simulink model "VINS"  (R2018a)
settings: Solver=FixedStepDiscrete  StartTime=0.0  StopTime=inf  FixedStep=1/Fs  RelTol=1e-3  EnableMultiTasking=on
PreLoadFcn:
  | modelDef = getModelDef(calibrateSFMA);
  | 
  | %imuPar = getImuPar('lmvpUncalibrated');
  | 
  | timeMatchThreshold = 1000;
undefined symbols (not defined in the file or in its folder): beep, dejitter_on, Fs, homogeneous3x4Transform_k_kmin1, imuLocationMm, imuPar, numStates, simData, tstamp_k_us, tstamp_kmin1_us
libraries: simulink x69, dspmtrx3 x35, dspindex x9, vrlib x7, dspstat3 x7, dspinverses x6, dspsigops x5, dspmathops x2, rtwdemowidgets x1, dspfactors x1, simulink_extras x1
(part 2 of 6)

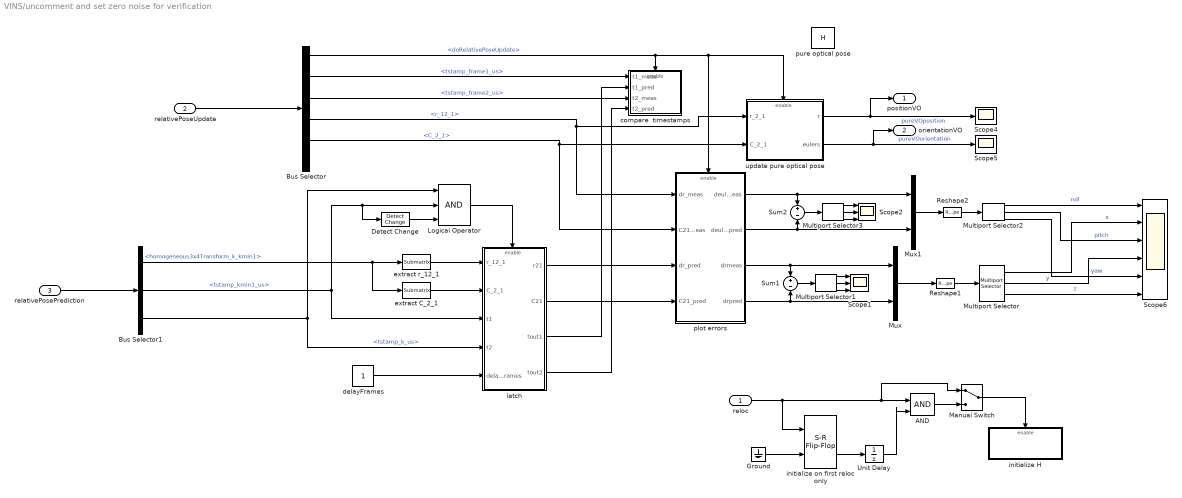
== system VINS/uncomment and set zero noise for verification ==
  reloc : Inport
  relativePoseUpdate : Inport  Port=2
  relativePosePrediction : Inport  Port=3
  AND : Logic  IconShape=distinctive  AllPortsSameDT=off  OutDataTypeStr=boolean
  Bus Selector : BusSelector  OutputSignals=doRelativePoseUpdate,tstamp_frame1_us,tstamp_frame2_us,r_12_1,C_2_1,poseErrorCovariance
  Bus Selector1 : BusSelector  OutputSignals=homogeneous3x4Transform_k_kmin1,tstamp_kmin1_us,tstamp_k_us
  Detect Change : simulink/Logic and Bit Operations/Detect Change  vinit=0  OutDataTypeStr=boolean
  Ground : Ground
  Logical Operator : Logic  Inputs=3  AllPortsSameDT=off  OutDataTypeStr=boolean
  Manual Switch : ManualSwitch
  Multiport Selector{,1..3} (4 alike) : dspindex/Multiport Selector  rowsOrCols=Rows  idxCellArray={1,2,3 }  idxErrMode=Clip Index
  Mux : Mux  Inputs=2
  Mux1 : Mux  Inputs=2
  Reshape1 : Reshape  OutputDimensionality=Customize  OutputDimensions=[3,2]
  Reshape2 : Reshape  OutputDimensionality=Customize  OutputDimensions=[3,2]
  Scope1 : Scope  NumInputPorts=3
  Scope2 : Scope  NumInputPorts=3
  Scope4 : Scope
  Scope5 : Scope
  Scope6 : Scope  NumInputPorts=6
  Sum1 : Sum  Inputs=+-
  Sum2 : Sum  Inputs=+-
  Unit Delay : UnitDelay  SampleTime=-1
  compare  timestamps : Subsystem  TreatAsAtomicUnit=on
  delayFrames : Constant
  extract C_2_1 : dspmtrx3/Submatrix  RowSpan=Range of rows  RowStartMode=First  RowStartIndex=1  RowEndMode=Index  RowEndIndex=3  ColSpan=Range of columns  ColStartMode=First  ColStartIndex=1  ColEndMode=Index  ColEndIndex=3
  extract r_12_1 : dspmtrx3/Submatrix  RowSpan=Range of rows  RowStartMode=First  RowStartIndex=1  RowEndMode=Index  RowEndIndex=3  ColSpan=One column  ColStartMode=Last  ColStartIndex=1  ColEndMode=Index  ColEndIndex=3
  initialize H : Subsystem  TreatAsAtomicUnit=on
  initialize on first reloc only : simulink_extras/Flip Flops/S-R Flip-Flop  initial_condition=0
  latch : Subsystem  TreatAsAtomicUnit=on
  plot errors : Subsystem  TreatAsAtomicUnit=on
  pure optical pose : DataStoreMemory  DataStoreName=H  ReadBeforeWriteMsg=warning  WriteAfterWriteMsg=warning  WriteAfterReadMsg=warning  InitialValue=eye(4)  ShowAdditionalParam=off
  update pure optical pose : Subsystem  TreatAsAtomicUnit=on
  positionVO : Outport
  orientationVO : Outport  Port=2
  wires:
  relativePoseUpdate/1 -> Bus Selector/1
  Bus Selector/1 -> plot errors/Enable, update pure optical pose/Enable, compare  timestamps/Enable  "<doRelativePoseUpdate>"
  Bus Selector/4 -> update pure optical pose/1(r_2_1), plot errors/1(dr_meas)  "<r_12_1>"
  Bus Selector/5 -> plot errors/2(C21_meas), update pure optical pose/2(C_2_1)  "<C_2_1>"
  relativePosePrediction/1 -> Bus Selector1/1
  Bus Selector1/1 -> extract C_2_1/1, extract r_12_1/1  "<homogeneous3x4Transform_k_kmin1>"
  Bus Selector/2 -> compare  timestamps/1(t1_meas)  "<tstamp_frame1_us>"
  Bus Selector/3 -> compare  timestamps/3(t2_meas)  "<tstamp_frame2_us>"
  extract r_12_1/1 -> latch/1(r_12_1)
  extract C_2_1/1 -> latch/2(C_2_1)
  Bus Selector1/3 -> latch/4(t2), Logical Operator/1  "<tstamp_k_us>"
  Bus Selector1/2 -> latch/3(t1), Detect Change/1, Logical Operator/2  "<tstamp_kmin1_us>"
  Logical Operator/1 -> latch/Enable
  latch/3(tout1) -> compare  timestamps/2(t1_pred)
  latch/4(tout2) -> compare  timestamps/4(t2_pred)
  latch/1(r21) -> plot errors/3(dr_pred)
  latch/2(C21) -> plot errors/4(C21_pred)
  plot errors/4(drpred) -> Mux/2, Sum1/2
  plot errors/3(drmeas) -> Mux/1, Sum1/1
  Sum1/1 -> Multiport Selector1/1
  delayFrames/1 -> latch/5(delayFrames)
  Detect Change/1 -> Logical Operator/3
  update pure optical pose/1(r) -> Scope4/1, positionVO/1  "pureVOposition"
  update pure optical pose/2(eulers) -> orientationVO/1, Scope5/1  "pureVOorientation"
  Mux/1 -> Reshape1/1
  Reshape1/1 -> Multiport Selector/1
  Multiport Selector1/3 -> Scope1/3
  Multiport Selector1/1 -> Scope1/1
  Multiport Selector1/2 -> Scope1/2
  Multiport Selector3/2 -> Scope2/2
  Multiport Selector3/1 -> Scope2/1
  Multiport Selector3/3 -> Scope2/3
  Reshape2/1 -> Multiport Selector2/1
  Mux1/1 -> Reshape2/1
  Sum2/1 -> Multiport Selector3/1
  plot errors/1(deul_meas) -> Sum2/1, Mux1/1
  plot errors/2(deul_pred) -> Sum2/2, Mux1/2
  Multiport Selector2/1 -> Scope6/1  "roll"
  Multiport Selector/1 -> Scope6/2  "x"
  Multiport Selector2/2 -> Scope6/3  "pitch"
  Multiport Selector/2 -> Scope6/4  "y"
  Multiport Selector2/3 -> Scope6/5  "yaw"
  Multiport Selector/3 -> Scope6/6  "z"
  reloc/1 -> initialize on first reloc only/1, Manual Switch/1, AND/1
  Manual Switch/1 -> initialize H/Enable
  initialize on first reloc only/2 -> Unit Delay/1
  Unit Delay/1 -> AND/2
  Ground/1 -> initialize on first reloc only/2
  AND/1 -> Manual Switch/2

== system VINS/INS/DT police ==
  In1 : Inport
  Data Store Read : DataStoreRead  DataStoreName=DataTypeRef
  Data Type Duplicate : DataTypeDuplicate
  wires:
  Data Store Read/1 -> Data Type Duplicate/1
  In1/1 -> Data Type Duplicate/2

== system VINS/augmentState/DT convert ==
  In1 : Inport
  Data Store Read : DataStoreRead  DataStoreName=DataTypeRef
  Data Type Conversion Inherited : simulink/Signal Attributes/Data Type Conversion Inherited  ConvertRealWorld=Real World Value  DoSatur=off
      settings: SourceProductName=Simulink  SourceProductBaseCode=SL
  Out1 : Outport
  wires:
  Data Type Conversion Inherited/1 -> Out1/1
  Data Store Read/1 -> Data Type Conversion Inherited/1
  In1/1 -> Data Type Conversion Inherited/2

== system VINS/augmentState/DT convert1 ==
  In1 : Inport
  Data Store Read : DataStoreRead  DataStoreName=DataTypeRef
  Data Type Conversion Inherited : simulink/Signal Attributes/Data Type Conversion Inherited  ConvertRealWorld=Real World Value  DoSatur=off
      settings: SourceProductName=Simulink  SourceProductBaseCode=SL
  Out1 : Outport
  wires:
  In1/1 -> Data Type Conversion Inherited/2
  Data Store Read/1 -> Data Type Conversion Inherited/1
  Data Type Conversion Inherited/1 -> Out1/1

== system VINS/augmentState/DT police1 ==
  In1 : Inport
  Data Store Read : DataStoreRead  DataStoreName=DataTypeRef
  Data Type Duplicate : DataTypeDuplicate
  wires:
  Data Store Read/1 -> Data Type Duplicate/1
  In1/1 -> Data Type Duplicate/2

== system VINS/augmentState/DT police2 ==
  In1 : Inport
  Data Store Read : DataStoreRead  DataStoreName=DataTypeRef
  Data Type Duplicate : DataTypeDuplicate
  wires:
  Data Store Read/1 -> Data Type Duplicate/1
  In1/1 -> Data Type Duplicate/2

== system VINS/augmentState/DT police3 ==
  In1 : Inport
  Data Store Read : DataStoreRead  DataStoreName=DataTypeRef
  Data Type Duplicate : DataTypeDuplicate
  wires:
  In1/1 -> Data Type Duplicate/2
  Data Store Read/1 -> Data Type Duplicate/1

== system VINS/augmentState/DT police4 ==
  In1 : Inport
  Data Store Read : DataStoreRead  DataStoreName=DataTypeRef
  Data Type Duplicate : DataTypeDuplicate
  wires:
  Data Store Read/1 -> Data Type Duplicate/1
  In1/1 -> Data Type Duplicate/2

== system VINS/augmentState/DT police5 ==
  In1 : Inport
  Data Store Read : DataStoreRead  DataStoreName=DataTypeRef
  Data Type Duplicate : DataTypeDuplicate
  wires:
  In1/1 -> Data Type Duplicate/2
  Data Store Read/1 -> Data Type Duplicate/1

== system VINS/augmentState/DT police6 ==
  In1 : Inport
  Data Store Read : DataStoreRead  DataStoreName=DataTypeRef
  Data Type Duplicate : DataTypeDuplicate
  wires:
  Data Store Read/1 -> Data Type Duplicate/1
  In1/1 -> Data Type Duplicate/2

== system VINS/augmentState/DT police7 ==
  In1 : Inport
  Data Store Read : DataStoreRead  DataStoreName=DataTypeRef
  Data Type Duplicate : DataTypeDuplicate
  wires:
  In1/1 -> Data Type Duplicate/2
  Data Store Read/1 -> Data Type Duplicate/1

== system VINS/augmentState/DT police8 ==
  In1 : Inport
  Data Store Read : DataStoreRead  DataStoreName=DataTypeRef
  Data Type Duplicate : DataTypeDuplicate
  wires:
  Data Store Read/1 -> Data Type Duplicate/1
  In1/1 -> Data Type Duplicate/2

== system VINS/augmentState/DT police9 ==
  In1 : Inport
  Data Store Read : DataStoreRead  DataStoreName=DataTypeRef
  Data Type Duplicate : DataTypeDuplicate
  wires:
  In1/1 -> Data Type Duplicate/2
  Data Store Read/1 -> Data Type Duplicate/1

== system VINS/augmentState/advancePoseIndex ==
  Bias : Bias  Bias=1
  Constant : Constant  Value=modelDef.maxNumDelayedPoses
  Data Store Read : DataStoreRead  DataStoreName=newestDelayedPoseIdx
  Data Store Write2 : DataStoreWrite  DataStoreName=newestDelayedPoseIdx
  Relational Operator : RelationalOperator  Operator=<=  OutDataTypeStr=boolean  RndMeth=Simplest
  Switch : Switch  Criteria=u2 > Threshold
  rollover back to one : Constant  Value=uint8(1)
  newIndex : Outport
  wires:
  Data Store Read/1 -> Bias/1
  Bias/1 -> Switch/1, Relational Operator/1
  Constant/1 -> Relational Operator/2
  Relational Operator/1 -> Switch/2
  Switch/1 -> newIndex/1, Data Store Write2/1  "newIndex"
  rollover back to one/1 -> Switch/3

== system VINS/calcDt/DT convert ==
  In1 : Inport
  Data Store Read : DataStoreRead  DataStoreName=DataTypeRef
  Data Type Conversion Inherited : simulink/Signal Attributes/Data Type Conversion Inherited  ConvertRealWorld=Real World Value  DoSatur=off
      settings: SourceProductName=Simulink  SourceProductBaseCode=SL
  Out1 : Outport
  wires:
  Data Type Conversion Inherited/1 -> Out1/1
  Data Store Read/1 -> Data Type Conversion Inherited/1
  In1/1 -> Data Type Conversion Inherited/2

== system VINS/cameraRelativePosePrediction/b frame to c frame ==
  Cbn : Inport
  r_nb_n : Inport  Port=2
  Enable : EnablePort
  Data Store Read5 : DataStoreRead  DataStoreName=r_bc_b
  Data Store Read9 : DataStoreRead  DataStoreName=Ccb
  Matrix Multiply : Product  Multiplication=Matrix(*)
  Matrix Multiply1 : Product  Multiplication=Matrix(*)
  Sum : Sum  Inputs=|++
  Ccn : Outport
  rcn : Outport  Port=2
  wires:
  Data Store Read9/1 -> Matrix Multiply1/2
  Matrix Multiply1/1 -> Ccn/1
  r_nb_n/1 -> Sum/1
  Matrix Multiply/1 -> Sum/2  "r_bc_n"
  Cbn/1 -> Matrix Multiply/1, Matrix Multiply1/1
  Data Store Read5/1 -> Matrix Multiply/2
  Sum/1 -> rcn/1  "r_nc_n"

== system VINS/cameraRelativePosePrediction/b frame to c frame1 ==
  Cbn : Inport
  r_nb_n : Inport  Port=2
  Enable : EnablePort
  Data Store Read5 : DataStoreRead  DataStoreName=r_bc_b
  Data Store Read9 : DataStoreRead  DataStoreName=Ccb
  Matrix Multiply : Product  Multiplication=Matrix(*)
  Matrix Multiply1 : Product  Multiplication=Matrix(*)
  Sum : Sum  Inputs=|++
  Ccn : Outport
  rcn : Outport  Port=2
  wires:
  Sum/1 -> rcn/1  "r_nc_n"
  Data Store Read5/1 -> Matrix Multiply/2
  Cbn/1 -> Matrix Multiply1/1, Matrix Multiply/1
  Matrix Multiply/1 -> Sum/2  "r_bc_n"
  r_nb_n/1 -> Sum/1
  Matrix Multiply1/1 -> Ccn/1
  Data Store Read9/1 -> Matrix Multiply1/2

== system VINS/cameraRelativePosePrediction/frameToFramePrediction ==
  Ccn_k : Inport
  r_nc_n_k : Inport  Port=2
  Ccn_kmin1 : Inport  Port=3
  r_nc_n_kmin1 : Inport  Port=4
  tstamp_vidcap_us : Inport  Port=5
  Enable : EnablePort
  Bus Creator : BusCreator  Inputs=homogeneous3x4Transform_k_kmin1,tstamp_k_us,tstamp_kmin1_us  OutDataTypeStr=Bus: cameraRelativePosePrediction  NonVirtualBus=on
  Data Type Conversion : DataTypeConversion
  Gain : Gain  Gain=1e-6
  MATLAB Function3 : MATLAB Function  TreatAsAtomicUnit=on
  Matrix Concatenate : Concatenate  Mode=Multidimensional array  ConcatenateDimension=2
  Matrix Multiply : Product  Multiplication=Matrix(*)
  Matrix Multiply1 : Product  Multiplication=Matrix(*)
  Permute Dimensions : PermuteDimensions
  Product : Product  Inputs=*/
  Scope1 : Scope
  Scope2 : Scope
  Scope3 : Scope
  Sum : Sum  Inputs=|+-
  Sum1 : Sum  Inputs=+-
  Unit Delay : UnitDelay  SampleTime=-1
  cameraRelativePosePrediction : Outport
  wires:
  Ccn_k/1 -> Matrix Multiply/2  "C_k_n"
  r_nc_n_k/1 -> Sum/1
  Ccn_kmin1/1 -> Permute Dimensions/1  "C_kmin1_n"
  Permute Dimensions/1 -> Matrix Multiply1/1, Matrix Multiply/1  "C_n_kmin1"
  r_nc_n_kmin1/1 -> Sum/2
  Sum/1 -> Matrix Multiply1/2
  Matrix Multiply/1 -> MATLAB Function3/1(Cbn), Matrix Concatenate/1  "C_k_kmin1"
  Matrix Multiply1/1 -> Product/1, Scope1/1, Matrix Concatenate/2  "r_k_kmin1"
  Matrix Concatenate/1 -> Data Type Conversion/1
  Bus Creator/1 -> cameraRelativePosePrediction/1
  Data Type Conversion/1 -> Bus Creator/1  "homogeneous3x4Transform_k_kmin1"
  tstamp_vidcap_us/1 -> Sum1/1, Bus Creator/2, Unit Delay/1  "tstamp_k_us"
  Unit Delay/1 -> Sum1/2, Bus Creator/3  "tstamp_kmin1_us"
  MATLAB Function3/1(eul) -> Scope2/1
  Sum1/1 -> Gain/1
  Product/1 -> Scope3/1
  Gain/1 -> Product/2

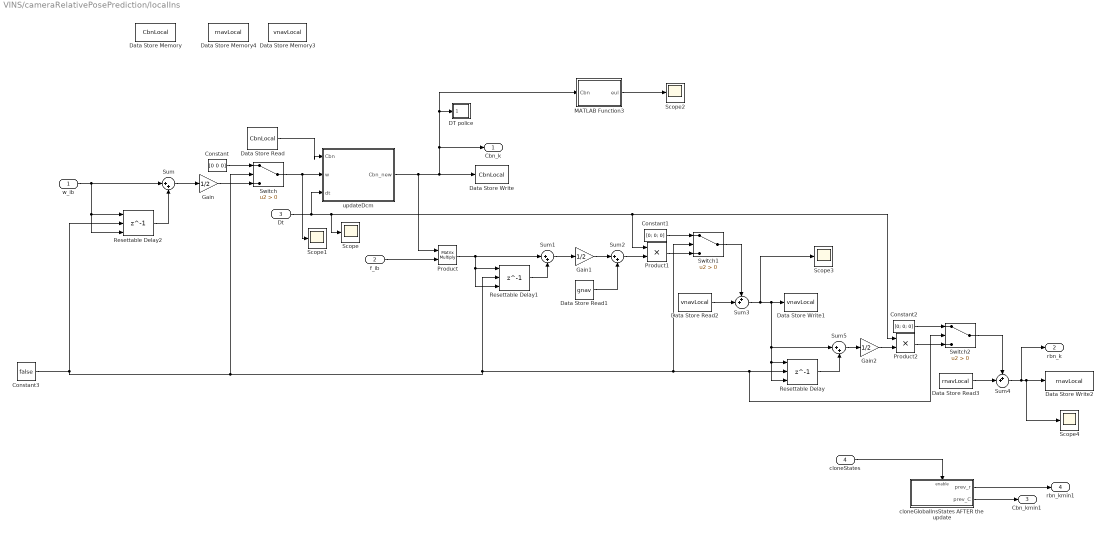
== system VINS/cameraRelativePosePrediction/localIns ==
  w_ib : Inport
  f_ib : Inport  Port=2
  Dt : Inport  Port=3
  cloneStates : Inport  Port=4
  Constant : Constant  Value=[0 0 0]
  Constant1 : Constant  Value=[0; 0; 0]  VectorParams1D=off  OutDataTypeStr=Inherit: Inherit via back propagation
  Constant2 : Constant  Value=[0; 0; 0]  VectorParams1D=off  OutDataTypeStr=Inherit: Inherit via back propagation
  Constant3 : Constant  Value=false
  DT police : Subsystem  TreatAsAtomicUnit=on
  Data Store Memory : DataStoreMemory  DataStoreName=CbnLocal  ReadBeforeWriteMsg=warning  WriteAfterWriteMsg=warning  WriteAfterReadMsg=warning  InitialValue=eye(3)  VectorParams1D=off  ShowAdditionalParam=off
  Data Store Memory3 : DataStoreMemory  DataStoreName=vnavLocal  ReadBeforeWriteMsg=warning  WriteAfterWriteMsg=warning  WriteAfterReadMsg=warning  InitialValue=[0;0;0]  VectorParams1D=off  ShowAdditionalParam=off
  Data Store Memory4 : DataStoreMemory  DataStoreName=rnavLocal  ReadBeforeWriteMsg=warning  WriteAfterWriteMsg=warning  WriteAfterReadMsg=warning  InitialValue=[0;0;0]  VectorParams1D=off  ShowAdditionalParam=off
  Data Store Read : DataStoreRead  DataStoreName=CbnLocal
  Data Store Read1 : DataStoreRead  DataStoreName=gnav
  Data Store Read2 : DataStoreRead  DataStoreName=vnavLocal
  Data Store Read3 : DataStoreRead  DataStoreName=rnavLocal
  Data Store Write : DataStoreWrite  DataStoreName=CbnLocal
  Data Store Write1 : DataStoreWrite  DataStoreName=vnavLocal
  Data Store Write2 : DataStoreWrite  Priority=1  DataStoreName=rnavLocal
  Gain : Gain  Gain=1/2
  Gain1 : Gain  Gain=1/2
  Gain2 : Gain  Gain=1/2
  MATLAB Function3 : MATLAB Function  TreatAsAtomicUnit=on
  Product : Product  Multiplication=Matrix(*)
  Product1 : Product
  Product2 : Product
  Resettable Delay : Delay  DelayLength=1  InitialConditionSource=Input port  ExternalReset=Level hold
      settings: InputPortMap=u0,r5,p4
  Resettable Delay1 : Delay  DelayLength=1  InitialConditionSource=Input port  ExternalReset=Level hold
      settings: InputPortMap=u0,r5,p4
  Resettable Delay2 : Delay  DelayLength=1  InitialConditionSource=Input port  ExternalReset=Level hold
      settings: InputPortMap=u0,r5,p4
  Scope{,1..4} (5 alike) : Scope
  Sum{,1..2,5} (4 alike) : Sum  Inputs=|++
  Sum3 : Sum  Inputs=++|
  Sum4 : Sum  Inputs=++|
  Switch : Switch  Criteria=u2 > Threshold
  Switch1 : Switch  Criteria=u2 > Threshold
  Switch2 : Switch  Criteria=u2 > Threshold
  cloneGlobalInsStates AFTER the update : Subsystem  Priority=2  TreatAsAtomicUnit=on
  updateDcm : MATLAB Function  TreatAsAtomicUnit=on
  Cbn_k : Outport
  rbn_k : Outport  Port=2
  Cbn_kmin1 : Outport  Port=3
  rbn_kmin1 : Outport  Port=4
  wires:
  Resettable Delay1/1 -> Sum1/2
  Resettable Delay/1 -> Sum5/2
  Gain2/1 -> Product2/2
  Sum3/1 -> Scope3/1, Data Store Write1/1, Sum5/1, Resettable Delay/1, Resettable Delay/3
  Sum5/1 -> Gain2/1
  Sum4/1 -> rbn_k/1, Scope4/1, Data Store Write2/1
  Data Store Read3/1 -> Sum4/2
  Switch1/1 -> Sum3/1
  Data Store Read2/1 -> Sum3/2
  Gain1/1 -> Sum2/1
  Sum1/1 -> Gain1/1
  Product/1 -> Sum1/1, Resettable Delay1/1, Resettable Delay1/3
  Sum2/1 -> Product1/2
  Data Store Read1/1 -> Sum2/2
  f_ib/1 -> Product/2
  Sum/1 -> Gain/1
  Resettable Delay2/1 -> Sum/2
  Data Store Read/1 -> updateDcm/1(Cbn)
  w_ib/1 -> Sum/1, Resettable Delay2/3, Resettable Delay2/1
  Dt/1 -> updateDcm/3(dt), Scope/1, Product1/1, Product2/1
  Constant3/1 -> Switch/2, Switch1/2, Switch2/2, Resettable Delay/2, Resettable Delay1/2, Resettable Delay2/2
  Gain/1 -> Switch/3
  Constant/1 -> Switch/1
  Product1/1 -> Switch1/3
  Constant1/1 -> Switch1/1
  Product2/1 -> Switch2/3
  Switch2/1 -> Sum4/1
  Constant2/1 -> Switch2/1
  Switch/1 -> updateDcm/2(w), Scope1/1
  cloneStates/1 -> cloneGlobalInsStates AFTER the update/Enable
  MATLAB Function3/1(eul) -> Scope2/1
  cloneGlobalInsStates AFTER the update/2(prev_C) -> Cbn_kmin1/1
  cloneGlobalInsStates AFTER the update/1(prev_r) -> rbn_kmin1/1
  updateDcm/1(Cbn_new) -> Cbn_k/1, MATLAB Function3/1(Cbn), DT police/1(In1), Data Store Write/1, Product/1

== system VINS/initStatesCovariances/DT police ==
  In1 : Inport
  Data Store Read : DataStoreRead  DataStoreName=DataTypeRef
  Data Type Duplicate : DataTypeDuplicate
  wires:
  Data Store Read/1 -> Data Type Duplicate/1
  In1/1 -> Data Type Duplicate/2

== system VINS/initStatesCovariances/initialize r_bc_b ==
  Enable : EnablePort
  Constant : Constant  Value=imuLocationMm  OutDataTypeStr=Inherit: Inherit via back propagation
  DT police : Subsystem  TreatAsAtomicUnit=on
  Data Store Write : DataStoreWrite  DataStoreName=r_bc_b
  Data Store Write1 : DataStoreWrite  DataStoreName=rnav
  Gain : Gain  Gain=-1/1000
  Gain1 : Gain  Gain=1/1000
  wires:
  Constant/1 -> Gain1/1, Gain/1
  Gain/1 -> DT police/1(In1), Data Store Write/1
  Gain1/1 -> Data Store Write1/1

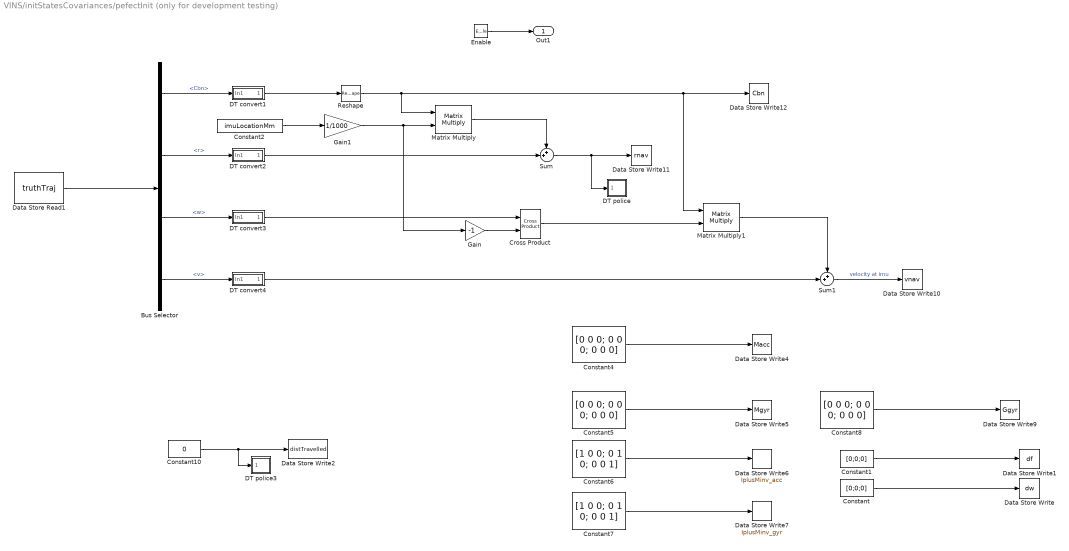
== system VINS/initStatesCovariances/pefectInit (only for development testing) ==
  Enable : EnablePort  ShowOutputPort=on
  Bus Selector : BusSelector  OutputSignals=Cbn,r,w,v
  Constant : Constant  Value=[0;0;0]  OutDataTypeStr=Inherit: Inherit via back propagation
  Constant1 : Constant  Value=[0;0;0]  OutDataTypeStr=Inherit: Inherit via back propagation
  Constant10 : Constant  Value=0  OutDataTypeStr=Inherit: Inherit via back propagation
  Constant2 : Constant  Value=imuLocationMm  OutDataTypeStr=Inherit: Inherit via back propagation
  Constant4 : Constant  Value=[0 0 0; 0 0 0; 0 0 0]  VectorParams1D=off  OutDataTypeStr=Inherit: Inherit via back propagation
  Constant5 : Constant  Value=[0 0 0; 0 0 0; 0 0 0]  VectorParams1D=off  OutDataTypeStr=Inherit: Inherit via back propagation
  Constant6 : Constant  Value=[1 0 0; 0 1 0; 0 0 1]  VectorParams1D=off  OutDataTypeStr=Inherit: Inherit via back propagation
  Constant7 : Constant  Value=[1 0 0; 0 1 0; 0 0 1]  VectorParams1D=off  OutDataTypeStr=Inherit: Inherit via back propagation
  Constant8 : Constant  Value=[0 0 0; 0 0 0; 0 0 0]  VectorParams1D=off  OutDataTypeStr=Inherit: Inherit via back propagation
  Cross Product : vrlib/Utilities/Cross Product
      settings: SourceProductBaseCode=VR
  DT convert1 : Subsystem
  DT convert2 : Subsystem
  DT convert3 : Subsystem
  DT convert4 : Subsystem
  DT police : Subsystem  TreatAsAtomicUnit=on
  DT police3 : Subsystem  TreatAsAtomicUnit=on
  Data Store Read1 : DataStoreRead  DataStoreName=truthTraj  DataStoreElements=truthTraj
  Data Store Write : DataStoreWrite  DataStoreName=dw
  Data Store Write1 : DataStoreWrite  DataStoreName=df
  Data Store Write10 : DataStoreWrite  DataStoreName=vnav
  Data Store Write11 : DataStoreWrite  DataStoreName=rnav
  Data Store Write12 : DataStoreWrite  DataStoreName=Cbn
  Data Store Write2 : DataStoreWrite  DataStoreName=distTravelled
  Data Store Write4 : DataStoreWrite  DataStoreName=Macc
  Data Store Write5 : DataStoreWrite  DataStoreName=Mgyr
  Data Store Write6 : DataStoreWrite  DataStoreName=IplusMinv_acc
  Data Store Write7 : DataStoreWrite  DataStoreName=IplusMinv_gyr
  Data Store Write9 : DataStoreWrite  DataStoreName=Ggyr
  Gain : Gain  Gain=-1
  Gain1 : Gain  Gain=1/1000
  Matrix Multiply : Product  Multiplication=Matrix(*)
  Matrix Multiply1 : Product  Multiplication=Matrix(*)
  Reshape : Reshape  OutputDimensionality=Customize  OutputDimensions=[3,3]
  Sum : Sum  Inputs=++|
  Sum1 : Sum  Inputs=++|
  Out1 : Outport  OutputWhenDisabled=reset  InitialOutput=false
  wires:
  Constant/1 -> Data Store Write/1
  Constant1/1 -> Data Store Write1/1
  Constant4/1 -> Data Store Write4/1
  Constant5/1 -> Data Store Write5/1
  Constant6/1 -> Data Store Write6/1
  Constant7/1 -> Data Store Write7/1
  Enable/1 -> Out1/1
  Constant8/1 -> Data Store Write9/1
  Data Store Read1/1 -> Bus Selector/1
  Bus Selector/2 -> DT convert2/1(In1)  "<r>"
  Bus Selector/1 -> DT convert1/1(In1)  "<Cbn>"
  Constant2/1 -> Gain1/1
  Gain/1 -> Cross Product/2
  Bus Selector/3 -> DT convert3/1(In1)  "<w>"
  Matrix Multiply/1 -> Sum/1
  Bus Selector/4 -> DT convert4/1(In1)  "<v>"
  Sum1/1 -> Data Store Write10/1  "velocity at imu"
  Sum/1 -> DT police/1(In1), Data Store Write11/1
  Matrix Multiply1/1 -> Sum1/1
  Cross Product/1 -> Matrix Multiply1/2
  Reshape/1 -> Matrix Multiply/1, Data Store Write12/1, Matrix Multiply1/1
  DT convert1/1(Out1) -> Reshape/1
  DT convert2/1(Out1) -> Sum/2
  DT convert3/1(Out1) -> Cross Product/1
  DT convert4/1(Out1) -> Sum1/2
  Constant10/1 -> DT police3/1(In1), Data Store Write2/1
  Gain1/1 -> Gain/1, Matrix Multiply/2

== system VINS/initStatesCovariances/realInit ==
  f_ib_b : Inport
  Enable : EnablePort  ShowOutputPort=on
  calcCbn : Subsystem  TreatAsAtomicUnit=on
  setStates : Subsystem  TreatAsAtomicUnit=on
  Out1 : Outport
  wires:
  calcCbn/1(Out1) -> setStates/Enable
  f_ib_b/1 -> calcCbn/1(f^b)
  calcCbn/2(Cbn) -> setStates/1(Cbn)
  setStates/1(Out1) -> Out1/1
  Enable/1 -> calcCbn/Enable

== system VINS/initStatesCovariances/setInitializedFlag ==
  Enable : EnablePort  ShowOutputPort=on
  Constant : Constant  Value=true
  Data Store Write : DataStoreWrite  DataStoreName=INITIALIZED
  Out1 : Outport  OutputWhenDisabled=reset  InitialOutput=false
  wires:
  Enable/1 -> Out1/1
  Constant/1 -> Data Store Write/1

== system VINS/initStatesCovariances/setP ==
  perfectInit : Inport
  Enable : EnablePort  ShowOutputPort=on
  Constant : Constant  Value=zeros(modelDef.numStates, modelDef.statesPerDelayedPose*modelDef.maxNumDelayedPoses)  OutDataTypeStr=Inherit: Inherit via back propagation
  Constant1 : Constant  Value=zeros(modelDef.statesPerDelayedPose*modelDef.maxNumDelayedPoses, modelDef.statesPerDelayedPose*modelDef.maxNumDelayedPoses)  OutDataTypeStr=Inherit: Inherit via back propagation
  DT police1 : Subsystem  TreatAsAtomicUnit=on
  DT police2 : Subsystem  TreatAsAtomicUnit=on
  DT police3 : Subsystem  TreatAsAtomicUnit=on
  Data Store Write : DataStoreWrite  DataStoreName=Pxx
  Data Store Write1 : DataStoreWrite  DataStoreName=Pxc
  Data Store Write2 : DataStoreWrite  DataStoreName=Pcc
  Environment Controller : simulink/Signal Routing/Environment Controller
      settings: SourceProductName=Simulink  SourceProductBaseCode=SL
  Environment Controller1 : simulink/Signal Routing/Environment Controller
      settings: SourceProductName=Simulink  SourceProductBaseCode=SL
  MATLAB Function1 : MATLAB Function  TreatAsAtomicUnit=on
  Switch : Switch  Criteria=u2 > Threshold
  Switch1 : Switch  Criteria=u2 > Threshold
  "initial position error, m rms" : Constant  Value=[0.01; 0.01; 0.01]  VectorParams1D=off  OutDataTypeStr=Inherit: Inherit via back propagation
  "initial position error, m rms1" : Constant  Value=[0.0; 0.0; 0.0]  VectorParams1D=off  OutDataTypeStr=Inherit: Inherit via back propagation
  "initial rotation error, rad rms" : Constant  Value=[0.1; 0.1; 0.1]  VectorParams1D=off  OutDataTypeStr=Inherit: Inherit via back propagation
  "initial rotation error, rad rms1" : Constant  Value=[0; 0; 0]  VectorParams1D=off  OutDataTypeStr=Inherit: Inherit via back propagation
  "initial rotation error, rad rms2" : Constant  Value=[0.1; 0.1; 0]  VectorParams1D=off  OutDataTypeStr=Inherit: Inherit via back propagation
  "initial vel error, m/s" : Constant  Value=[1; 1; 1]  VectorParams1D=off  OutDataTypeStr=Inherit: Inherit via back propagation
  "initial vel error, m/s1" : Constant  Value=[0.05; 0.05; 0.05]  VectorParams1D=off  OutDataTypeStr=Inherit: Inherit via back propagation
  Out1 : Outport  OutputWhenDisabled=reset  InitialOutput=false
  wires:
  Enable/1 -> Out1/1
  Environment Controller1/1 -> DT police2/1(In1), MATLAB Function1/2(initialPosUncert)
  Environment Controller/1 -> DT police1/1(In1), MATLAB Function1/1(initialRotUncert)
  MATLAB Function1/1(P0) -> Data Store Write/1
  Constant/1 -> Data Store Write1/1
  Constant1/1 -> Data Store Write2/1
  "initial rotation error, rad rms"/1 -> Environment Controller/2
  Switch/1 -> Environment Controller/1
  "initial position error, m rms"/1 -> Environment Controller1/2
  "initial position error, m rms1"/1 -> Environment Controller1/1
  Switch1/1 -> DT police3/1(In1), MATLAB Function1/3(initialVelUncert)
  "initial rotation error, rad rms2"/1 -> Switch/3
  perfectInit/1 -> Switch1/2, Switch/2
  "initial rotation error, rad rms1"/1 -> Switch/1
  "initial vel error, m/s"/1 -> Switch1/3
  "initial vel error, m/s1"/1 -> Switch1/1

== system VINS/measUpdate/DT convert ==
  In1 : Inport
  Data Store Read : DataStoreRead  DataStoreName=DataTypeRef
  Data Type Conversion Inherited : simulink/Signal Attributes/Data Type Conversion Inherited  ConvertRealWorld=Real World Value  DoSatur=off
      settings: SourceProductName=Simulink  SourceProductBaseCode=SL
  Out1 : Outport
  wires:
  Data Type Conversion Inherited/1 -> Out1/1
  Data Store Read/1 -> Data Type Conversion Inherited/1
  In1/1 -> Data Type Conversion Inherited/2

== system VINS/measUpdate/DT convert1 ==
  In1 : Inport
  Data Store Read : DataStoreRead  DataStoreName=DataTypeRef
  Data Type Conversion Inherited : simulink/Signal Attributes/Data Type Conversion Inherited  ConvertRealWorld=Real World Value  DoSatur=off
      settings: SourceProductName=Simulink  SourceProductBaseCode=SL
  Out1 : Outport
  wires:
  In1/1 -> Data Type Conversion Inherited/2
  Data Store Read/1 -> Data Type Conversion Inherited/1
  Data Type Conversion Inherited/1 -> Out1/1

== system VINS/measUpdate/DT convert2 ==
  In1 : Inport
  Data Store Read : DataStoreRead  DataStoreName=DataTypeRef
  Data Type Conversion Inherited : simulink/Signal Attributes/Data Type Conversion Inherited  ConvertRealWorld=Real World Value  DoSatur=off
      settings: SourceProductName=Simulink  SourceProductBaseCode=SL
  Out1 : Outport
  wires:
  Data Type Conversion Inherited/1 -> Out1/1
  Data Store Read/1 -> Data Type Conversion Inherited/1
  In1/1 -> Data Type Conversion Inherited/2

== system VINS/measUpdate/DT convert3 ==
  In1 : Inport
  Data Store Read : DataStoreRead  DataStoreName=DataTypeRef
  Data Type Conversion Inherited : simulink/Signal Attributes/Data Type Conversion Inherited  ConvertRealWorld=Real World Value  DoSatur=off
      settings: SourceProductName=Simulink  SourceProductBaseCode=SL
  Out1 : Outport
  wires:
  In1/1 -> Data Type Conversion Inherited/2
  Data Store Read/1 -> Data Type Conversion Inherited/1
  Data Type Conversion Inherited/1 -> Out1/1

== system VINS/measUpdate/DT convert4 ==
  In1 : Inport
  Data Store Read : DataStoreRead  DataStoreName=DataTypeRef
  Data Type Conversion Inherited : simulink/Signal Attributes/Data Type Conversion Inherited  ConvertRealWorld=Real World Value  DoSatur=off
      settings: SourceProductName=Simulink  SourceProductBaseCode=SL
  Out1 : Outport
  wires:
  Data Type Conversion Inherited/1 -> Out1/1
  Data Store Read/1 -> Data Type Conversion Inherited/1
  In1/1 -> Data Type Conversion Inherited/2

== system VINS/measUpdate/DT convert5 ==
  In1 : Inport
  Data Store Read : DataStoreRead  DataStoreName=DataTypeRef
  Data Type Conversion Inherited : simulink/Signal Attributes/Data Type Conversion Inherited  ConvertRealWorld=Real World Value  DoSatur=off
      settings: SourceProductName=Simulink  SourceProductBaseCode=SL
  Out1 : Outport
  wires:
  Data Type Conversion Inherited/1 -> Out1/1
  Data Store Read/1 -> Data Type Conversion Inherited/1
  In1/1 -> Data Type Conversion Inherited/2

== system VINS/measUpdate/DT convert6 ==
  In1 : Inport
  Data Store Read : DataStoreRead  DataStoreName=DataTypeRef
  Data Type Conversion Inherited : simulink/Signal Attributes/Data Type Conversion Inherited  ConvertRealWorld=Real World Value  DoSatur=off
      settings: SourceProductName=Simulink  SourceProductBaseCode=SL
  Out1 : Outport
  wires:
  In1/1 -> Data Type Conversion Inherited/2
  Data Store Read/1 -> Data Type Conversion Inherited/1
  Data Type Conversion Inherited/1 -> Out1/1

== system VINS/measUpdate/absolutePoseUpdate ==
  delayedPoseIdx : Inport
  innovation : Inport  Port=2
  R : Inport  Port=3
  Enable : EnablePort
  DT police : Subsystem  TreatAsAtomicUnit=on
  Data Store Read1 : DataStoreRead  DataStoreName=Pxc
  Data Store Read2 : DataStoreRead  DataStoreName=Pcc
  Data Store Read3 : DataStoreRead  DataStoreName=Pxx
  Demux : Demux  Outputs=2
  Extract Diagonal : dspmtrx3/Extract Diagonal
      settings: SourceProductName=DSP System Toolbox  SourceProductBaseCode=DS
  Logical Operator : Logic  Operator=NOT  Inputs=1  IconShape=distinctive  AllPortsSameDT=off  OutDataTypeStr=boolean
  Permute Dimensions : PermuteDimensions
  Product1 : Product  Multiplication=Matrix(*)
  Scope{,1,4,6} (4 alike) : Scope
  Sqrt : Sqrt  SaturateOnIntegerOverflow=on
  applyErrors : Subsystem
  calculateKalmanGain : MATLAB Function  TreatAsAtomicUnit=on
  "chi2 with 6dof, 95% less than 12.59" : simulink/Logic and Bit Operations/Compare To Constant  relop=<=  const=12.59  OutDataTypeStr=boolean
  dr : Selector  InputPortWidth=6  IndexOptions=Index vector (dialog)  Indices=[4 5 6]  OutputSizes=1
  formMeasurementMatrix : Subsystem
  get row indices : Subsystem  TreatAsAtomicUnit=on
  hcat : Concatenate  Mode=Multidimensional array  ConcatenateDimension=2
  hcat1 : Concatenate  Mode=Multidimensional array  ConcatenateDimension=2
  phi : Selector  InputPortWidth=6  IndexOptions=Index vector (dialog)  Indices=[1 2 3]  OutputSizes=1
  pos sigmas : Scope
  rot sigmas : Scope
  updateCovariance : Subsystem
  vcat : Concatenate  Mode=Multidimensional array
  measRejected : Outport  OutputWhenDisabled=reset  InitialOutput=0
  wires:
  dr/1 -> Scope1/1
  phi/1 -> Scope/1
  Product1/1 -> applyErrors/1(errors)  "errors"
  Data Store Read2/1 -> hcat1/2
  Permute Dimensions/1 -> hcat1/1  "Pcx"
  Data Store Read1/1 -> hcat/2, Permute Dimensions/1
  Data Store Read3/1 -> hcat/1
  hcat1/1 -> vcat/2
  hcat/1 -> vcat/1
  formMeasurementMatrix/1(Out1) -> DT police/1(In1), updateCovariance/2(H), calculateKalmanGain/2(H)
  innovation/1 -> calculateKalmanGain/4(nu), Product1/2, dr/1, phi/1
  vcat/1 -> updateCovariance/1(P), calculateKalmanGain/1(P)
  calculateKalmanGain/2(K) -> updateCovariance/3(K), Product1/1
  delayedPoseIdx/1 -> Scope4/1, get row indices/1(idx)
  get row indices/1(rows) -> formMeasurementMatrix/1(rows)
  R/1 -> Extract Diagonal/1, updateCovariance/4(R), calculateKalmanGain/3(R)
  Sqrt/1 -> Demux/1
  Demux/2 -> pos sigmas/1
  Demux/1 -> rot sigmas/1
  Extract Diagonal/1 -> Sqrt/1
  calculateKalmanGain/1(chiSquared) -> "chi2 with 6dof, 95% less than 12.59"/1, Scope6/1
  Logical Operator/1 -> measRejected/1
  "chi2 with 6dof, 95% less than 12.59"/1 -> updateCovariance/Enable, applyErrors/Enable, Logical Operator/1

== system VINS/measUpdate/commanded reloc ==
  imuSample : Inport
  Bus Selector1 : BusSelector  OutputSignals=jumpToXyz,xyz,jumpToYaw,yaw
  DT convert2 : Subsystem
  DT convert3 : Subsystem
  OR : Logic  Operator=OR  IconShape=distinctive  AllPortsSameDT=off  OutDataTypeStr=boolean
  setPosition1 : Subsystem  TreatAsAtomicUnit=on
  setYaw1 : Subsystem  TreatAsAtomicUnit=on
  reloc : Outport
  wires:
  Bus Selector1/2 -> DT convert2/1(In1)  "<xyz>"
  DT convert2/1(Out1) -> setPosition1/1(r_nc_n)
  imuSample/1 -> Bus Selector1/1
  Bus Selector1/4 -> DT convert3/1(In1)  "<yaw>"
  DT convert3/1(Out1) -> setYaw1/1(yaw)
  Bus Selector1/3 -> setYaw1/Enable, OR/2  "<jumpToYaw>"
  Bus Selector1/1 -> OR/1, setPosition1/Enable  "<jumpToXyz>"
  OR/1 -> reloc/1
  setYaw1/1(yawChanged) -> setPosition1/2(yawChanged)

== system VINS/measUpdate/compass meas update ==
  note: this is just to enforce block execution order
  In1 : Inport
  m^b : Inport  Port=2
  Enable : EnablePort
  Data Store Read1 : DataStoreRead  DataStoreName=Cbn
  Data Store Read3 : DataStoreRead  DataStoreName=Pxx
  Data Store Write : DataStoreWrite  DataStoreName=Pxx
  Demux : Demux  Outputs=3
  Gain : Gain  Gain=-1
  H : Constant  Value=[ 0 0 1]  VectorParams1D=off
  MATLAB Function1 : MATLAB Function  TreatAsAtomicUnit=on
  MATLAB Function3 : MATLAB Function  TreatAsAtomicUnit=on
  Product : Product  Multiplication=Matrix(*)
  Product1 : Product  Multiplication=Matrix(*)
  R assumes 10 deg rms compass noise : Constant  Value=0.34^2
  Scope : Scope
  Scope1 : Scope
  Scope2 : Scope
  Trigonometric Function : Trigonometry  Operator=atan2
  update the Cbn with the errors : Subsystem
  Out1 : Outport
  wires:
  Gain/1 -> Scope1/1, Product1/2
  H/1 -> MATLAB Function3/3(H), MATLAB Function1/2(H)
  Demux/1 -> Trigonometric Function/2
  Demux/2 -> Trigonometric Function/1
  In1/1 -> Out1/1
  Data Store Read1/1 -> Product/1  "Cbn hat"
  Product/1 -> Demux/1  "m^nhat"
  Trigonometric Function/1 -> Gain/1  "nu = 0 - psi"
  MATLAB Function1/2(K) -> Scope2/1, MATLAB Function3/2(K), Product1/1
  MATLAB Function3/1(Pplus) -> Data Store Write/1
  m^b/1 -> Product/2
  Data Store Read3/1 -> MATLAB Function3/1(P), MATLAB Function1/1(P)
  R assumes 10 deg rms compass noise/1 -> MATLAB Function3/4(R), MATLAB Function1/3(R)
  Product1/1 -> Scope/1, update the Cbn with the errors/1(phi  rotation errors)  "phi  rotation errors"

== system VINS/measUpdate/formDelayedInnovation ==
  idx : Inport
  r_nc_n : Inport  Port=2
  C_c_n_meas : Inport  Port=3
  Enable : EnablePort
  Ccn*Cbc*Cnbhat = I + phiX : Product  Inputs=3  Multiplication=Matrix(*)
  Data Store Read : DataStoreRead  DataStoreName=C_b_n_list
  Data Store Read1 : DataStoreRead  DataStoreName=r_b_n_list
  Data Store Read2 : DataStoreRead  DataStoreName=Ccb
  Data Store Read3 : DataStoreRead  DataStoreName=Cbn
  Data Store Read4 : DataStoreRead  DataStoreName=r_bc_b
  MATLAB Function3 : MATLAB Function  TreatAsAtomicUnit=on
  Matrix Multiply : Product  Multiplication=Matrix(*)
  Mux : Mux  Inputs=[3 3]
  Permute Dimensions : PermuteDimensions
  Permute Dimensions1 : PermuteDimensions
  Scope : Scope
  Scope1 : Scope
  Selector1 : Selector  NumberOfDimensions=3  InputPortWidth=3  IndexOptions=Index vector (dialog),Index vector (dialog),Index vector (port)  Indices=1:3,1:3,1  OutputSizes=1,1,1
  Selector3 : Selector  NumberOfDimensions=3  InputPortWidth=3  IndexOptions=Index vector (dialog),Index vector (dialog),Index vector (port)  Indices=1:3,1,1  OutputSizes=1,1,1
  Sum : Sum  Inputs=++|
  Sum1 : Sum  Inputs=-+|
  nu : Outport
  wires:
  Mux/1 -> nu/1
  Sum1/1 -> Mux/2, Scope1/1  "dr_nb_n"
  r_nc_n/1 -> Sum1/1
  Sum/1 -> Sum1/2  "r_nc_n_hat"
  Selector3/1 -> Sum/2  "r_nb_n_hat"
  MATLAB Function3/1(eul) -> Mux/1, Scope/1
  Ccn*Cbc*Cnbhat = I + phiX/1 -> MATLAB Function3/1(Cbn)
  Permute Dimensions/1 -> Ccn*Cbc*Cnbhat = I + phiX/3  "Cnbhat"
  Selector1/1 -> Permute Dimensions/1  "Cbnhat"
  C_c_n_meas/1 -> Ccn*Cbc*Cnbhat = I + phiX/1
  Data Store Read1/1 -> Selector3/1
  idx/1 -> Selector1/2, Selector3/2
  Data Store Read/1 -> Selector1/1
  Data Store Read2/1 -> Permute Dimensions1/1
  Matrix Multiply/1 -> Sum/1  "r_bc_n"
  Data Store Read3/1 -> Matrix Multiply/1
  Data Store Read4/1 -> Matrix Multiply/2
  Permute Dimensions1/1 -> Ccn*Cbc*Cnbhat = I + phiX/2  "Cbc"

== system VINS/measUpdate/get pose indices ==
  t1_us : Inport
  t2_us : Inport  Port=2
  Enable : EnablePort
  Compare To Constant : simulink/Logic and Bit Operations/Compare To Constant  relop===  const=1  OutDataTypeStr=boolean
  Compare To Constant1 : simulink/Logic and Bit Operations/Compare To Constant  relop===  const=1  OutDataTypeStr=boolean
  Constant : Constant  Value=uint32(0)
  Constant1 : Constant  Value=uint32(0)
  Data Store Read1 : DataStoreRead  DataStoreName=tstamp_list
  Display : Display
  Display1 : Display
  Display2 : Display
  Maximum : dspstat3/Maximum  operation=maximum  fcn=Index  indexBase=One  operateOver=Entire input  Dimension=1  InputProcessing=Columns as channels (frame based)  reset=None  roiEnable=off  roiType=Rectangles  roiPortion=Entire ROI  roiOutput=Individual statistics for each ROI  roiFlag=off  roundingMode=Floor  overflowMode=off  accumDataTypeStr=Inherit: Same as product output  accumLastDataTypeStr=Inherit: Same as product output
  Maximum1 : dspstat3/Maximum  operation=maximum  fcn=Index  indexBase=One  operateOver=Entire input  Dimension=1  InputProcessing=Columns as channels (frame based)  reset=None  roiEnable=off  roiType=Rectangles  roiPortion=Entire ROI  roiOutput=Individual statistics for each ROI  roiFlag=off  roundingMode=Floor  overflowMode=off  accumDataTypeStr=Inherit: Same as product output  accumLastDataTypeStr=Inherit: Same as product output
  Scope : Scope
  Scope1 : Scope
  Scope2 : Scope
  Sum : Sum  Inputs=+
  Sum1 : Sum  Inputs=+
  Sum2 : Sum  Inputs=+-|
  Switch : Switch  Criteria=u2 > Threshold
  Switch1 : Switch  Criteria=u2 > Threshold
  Unit Delay : UnitDelay  SampleTime=-1
  almostEqual : Subsystem
  almostEqual1 : Subsystem
  idx1 : Outport  OutputWhenDisabled=reset  InitialOutput=0
  idx2 : Outport  Port=2  OutputWhenDisabled=reset  InitialOutput=0
  wires:
  t2_us/1 -> Unit Delay/1, Display2/1, Sum2/1, almostEqual1/2(In2)
  Sum/1 -> Compare To Constant/1
  Compare To Constant/1 -> Scope/1, Switch/2
  Maximum/1 -> Switch/1
  Switch/1 -> idx1/1
  Constant/1 -> Switch/3
  Compare To Constant1/1 -> Scope1/1, Switch1/2
  Sum1/1 -> Compare To Constant1/1
  Maximum1/1 -> Switch1/1
  Constant1/1 -> Switch1/3
  almostEqual1/1(Out1) -> Sum1/1, Maximum1/1
  Switch1/1 -> idx2/1
  almostEqual/1(Out1) -> Sum/1, Maximum/1
  Data Store Read1/1 -> Display/1, almostEqual1/1(In1), almostEqual/1(In1)
  t1_us/1 -> Display1/1, almostEqual/2(In2)
  Unit Delay/1 -> Sum2/2
  Sum2/1 -> Scope2/1

== system VINS/measUpdate/get pose indices1 ==
  t_vidcap_us : Inport
  Enable : EnablePort
  Compare To Constant : simulink/Logic and Bit Operations/Compare To Constant  relop===  const=1  OutDataTypeStr=boolean
  Constant : Constant  Value=uint32(0)
  Data Store Read1 : DataStoreRead  DataStoreName=tstamp_list
  Maximum : dspstat3/Maximum  operation=maximum  fcn=Index  indexBase=One  operateOver=Entire input  Dimension=1  InputProcessing=Columns as channels (frame based)  reset=None  roiEnable=off  roiType=Rectangles  roiPortion=Entire ROI  roiOutput=Individual statistics for each ROI  roiFlag=off  roundingMode=Floor  overflowMode=off  accumDataTypeStr=Inherit: Same as product output  accumLastDataTypeStr=Inherit: Same as product output
  Sum : Sum  Inputs=+
  Switch : Switch  Criteria=u2 > Threshold
  almostEqual : Subsystem
  delayedPoseIdx : Outport  OutputWhenDisabled=reset  InitialOutput=0
  wires:
  Constant/1 -> Switch/3
  Switch/1 -> delayedPoseIdx/1
  Maximum/1 -> Switch/1
  Compare To Constant/1 -> Switch/2
  Sum/1 -> Compare To Constant/1
  almostEqual/1(Out1) -> Maximum/1, Sum/1
  t_vidcap_us/1 -> almostEqual/2(In2)
  Data Store Read1/1 -> almostEqual/1(In1)

== system VINS/measUpdate/gravity meas update ==
  note: this is just to enforce block execution order
  In1 : Inport
  f_ib^b : Inport  Port=2
  stilltime : Inport  Port=3
  Constant : Constant  Value=eye(3)
  Data Store Read1 : DataStoreRead  DataStoreName=Cbn
  Data Store Read3 : DataStoreRead  DataStoreName=Pxx
  Data Store Write : DataStoreWrite  DataStoreName=Pxx
  MATLAB Function1 : MATLAB Function  TreatAsAtomicUnit=on
  MATLAB Function2 : MATLAB Function  TreatAsAtomicUnit=on
  MATLAB Function3 : MATLAB Function  TreatAsAtomicUnit=on
  Math Function : Math  Operator=reciprocal  SaturateOnIntegerOverflow=on
  Math Function1 : Math  Operator=square  SaturateOnIntegerOverflow=on
  Pad : dspsigops/Pad  padAlong=Rows  dimsToPad=1  valSrc=Specify via dialog  padVal=0  spec=Output size  padNumOutRowsSpecMethod=User-specified  numOutRows=1  padNumOutColsSpecMethod=User-specified  numOutCols=numStates  isVarDimsMode=off  padBeginning=0  padEnd=0  outSizeMode=User-specified  outSize=1  padSigAt=End  trunc_flag=None  roundingMode=Floor  overflowMode=off  truncOrWrapMode=Truncate  wrap_flag=None
      settings: SourceProductName=DSP System Toolbox  SourceProductBaseCode=DS
  Permute Dimensions : PermuteDimensions
  Product : Product  Multiplication=Matrix(*)
  Product1 : Product  Multiplication=Matrix(*)
  Product2 : Product
  Product3 : Product  Multiplication=Matrix(*)
  Saturation : Saturate  UpperLimit=9.8*4  LowerLimit=1
  Sum1 : Sum  Inputs=|+-
  "specific force at rest is up, which is -z in NED frame" : Constant  Value=[ 0; 0; -9.8]
  update the Cbn and b_g with the errors : Subsystem
  Out1 : Outport
  wires:
  MATLAB Function1/2(K) -> MATLAB Function3/2(K), Product1/1
  Pad/1 -> MATLAB Function1/2(H), MATLAB Function3/3(H)
  Math Function1/1 -> Product2/2
  stilltime/1 -> Math Function/1
  Saturation/1 -> Math Function1/1
  Math Function/1 -> Saturation/1
  Constant/1 -> Product2/1
  Product1/1 -> update the Cbn and b_g with the errors/1(" error state estimates")  "errors"
  Product2/1 -> MATLAB Function1/3(R), MATLAB Function3/4(R)
  Data Store Read3/1 -> MATLAB Function1/1(P), MATLAB Function3/1(P)
  MATLAB Function2/1(res) -> Product3/2
  "specific force at rest is up, which is -z in NED frame"/1 -> Product/2, MATLAB Function2/1(inp_vr)
  Product3/1 -> Pad/1
  MATLAB Function3/1(Pplus) -> Data Store Write/1
  Sum1/1 -> Product1/2  "nu = z-zhat"
  Product/1 -> Sum1/2  "zhat"
  Permute Dimensions/1 -> Product/1, Product3/1  "Cnb hat"
  Data Store Read1/1 -> Permute Dimensions/1  "Cbn hat"
  f_ib^b/1 -> Sum1/1  "when still,  z = Cnb*[0 0 -9.8]' + v"
  In1/1 -> Out1/1

== system VINS/measUpdate/modeController ==
  Compare To Constant2 : simulink/Logic and Bit Operations/Compare To Constant  relop=<=  const=1.5*pi/180  OutDataTypeStr=boolean
  Data Store Read1 : DataStoreRead  DataStoreName=Pxx
  Extract Diagonal : dspmtrx3/Extract Diagonal
      settings: SourceProductName=DSP System Toolbox  SourceProductBaseCode=DS
  Maximum : dspstat3/Maximum  operation=maximum  fcn=Value  indexBase=One  operateOver=Entire input  Dimension=1  InputProcessing=Columns as channels (frame based)  reset=None  roiEnable=off  roiType=Rectangles  roiPortion=Entire ROI  roiOutput=Individual statistics for each ROI  roiFlag=off  roundingMode=Floor  overflowMode=off  accumDataTypeStr=Inherit: Same as product output  accumLastDataTypeStr=Inherit: Same as product output
  Sqrt : Sqrt  SaturateOnIntegerOverflow=on
  Submatrix : dspmtrx3/Submatrix  RowSpan=Range of rows  RowStartMode=First  RowStartIndex=1  RowEndMode=Index  RowEndIndex=2  ColSpan=Range of columns  ColStartMode=First  ColStartIndex=1  ColEndMode=Index  ColEndIndex=2
  set useRpus = true : Subsystem  Commented=on  TreatAsAtomicUnit=on
  wires:
  Maximum/1 -> Compare To Constant2/1
  Submatrix/1 -> Extract Diagonal/1
  Sqrt/1 -> Maximum/1
  Extract Diagonal/1 -> Sqrt/1
  Compare To Constant2/1 -> set useRpus = true/Enable
  Data Store Read1/1 -> Submatrix/1

== system VINS/measUpdate/opticalValid ==
  t_lastRpu_us : Inport
  vid_period : Inport  Port=2
  t_imu_us : Inport  Port=3
  DT convert1 : Subsystem
  Gain : Gain  Gain=3.1
  Gain2 : Gain  Gain=1e-6
  Relational Operator : RelationalOperator  Operator=<=  OutDataTypeStr=boolean  RndMeth=Simplest
  Sum : Sum  Inputs=|+-
  "opticalValid " : Outport
  wires:
  Gain2/1 -> DT convert1/1(In1)
  t_imu_us/1 -> Sum/1
  t_lastRpu_us/1 -> Sum/2
  Sum/1 -> Gain2/1
  DT convert1/1(Out1) -> Relational Operator/1
  vid_period/1 -> Gain/1
  Gain/1 -> Relational Operator/2
  Relational Operator/1 -> "opticalValid "/1

== system VINS/measUpdate/plotVidLatency ==
  tstamp_frame1_us : Inport
  tstamp_frame2_us : Inport  Port=2
  t_imu : Inport  Port=3
  Enable : EnablePort
  Compare To Constant : simulink/Logic and Bit Operations/Compare To Constant  relop=>=  const=modelDef.maxNumDelayedPoses  OutDataTypeStr=boolean
  Compare To Constant1 : simulink/Logic and Bit Operations/Compare To Constant  relop=<  const=0  OutDataTypeStr=boolean
  Constant : Constant
  DT convert : Subsystem
  DT convert1 : Subsystem
  DT convert2 : Subsystem
  Delay : Delay  DelayLength=1  InitialConditionSource=Input port
      settings: InputPortMap=u0,p4
  Gain1 : Gain  Gain=1e-6
  Gain2 : Gain  Gain=1e-6
  Gain3 : Gain  Gain=1e-6
  Logical Operator : Logic  AllPortsSameDT=off  OutDataTypeStr=boolean
  Median Filter : dspstat3/Median Filter  WindowLength=30  SimulateUsing=Code generation
      settings: SourceProductName=DSP System Toolbox  SourceProductBaseCode=DS
  Product : Product  Inputs=/*
  Scope : Scope
  Scope1 : Scope
  Scope2 : Scope
  Sum1 : Sum  Inputs=-+
  Sum2 : Sum  Inputs=-+
  Sum3 : Sum  Inputs=+-
  let median filter fill up : Delay  DelayLength=30
  newerFrameLatency : Scope
  olderFrameLatency : Scope
  set 0x08 bit : Subsystem  TreatAsAtomicUnit=on
  set 0x10 bit : Subsystem  TreatAsAtomicUnit=on
  t_imu_latched : Outport
  video period : Outport  Port=2
  wires:
  t_imu/1 -> t_imu_latched/1, Gain2/1
  tstamp_frame2_us/1 -> Gain3/1
  Sum2/1 -> Compare To Constant1/1, newerFrameLatency/1  "newer frame latency"
  Delay/1 -> Sum1/1
  Sum1/1 -> Scope2/1, Median Filter/1
  Product/1 -> Scope/1, Compare To Constant/1  "videoDelayFrames"
  Median Filter/1 -> Scope1/1, video period/1, Product/1
  Gain2/1 -> DT convert1/1(In1)
  Gain3/1 -> DT convert/1(In1)
  DT convert/1(Out1) -> Delay/1, Delay/2, Sum1/2, Sum2/1
  DT convert1/1(Out1) -> Sum3/1, Sum2/2
  Constant/1 -> let median filter fill up/1
  let median filter fill up/1 -> Logical Operator/2
  Logical Operator/1 -> set 0x08 bit/Enable
  Compare To Constant/1 -> Logical Operator/1
  Gain1/1 -> DT convert2/1(In1)
  tstamp_frame1_us/1 -> Gain1/1
  DT convert2/1(Out1) -> Sum3/2
  Sum3/1 -> Product/2, olderFrameLatency/1  "older frame latency"
  Compare To Constant1/1 -> set 0x10 bit/Enable
